simulink model "zawory_wyliczane"  (R2021b)
settings: Solver=VariableStepAuto  StartTime=0.0  StopTime=10.0  RelTol=1e-3
undefined symbols (not defined in the file): dpoN, dRz_b, dRz_g, dRz_p, Rb, Rg, Rk, Rp, RzN, skok_czas, zmiana_po
settings Model: Creator=adams  LastModifiedBy=adams

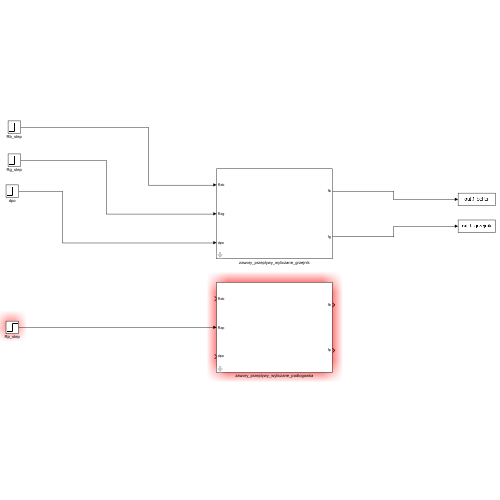
[thumbnail: Simulink's stored preview of the top-level diagram]
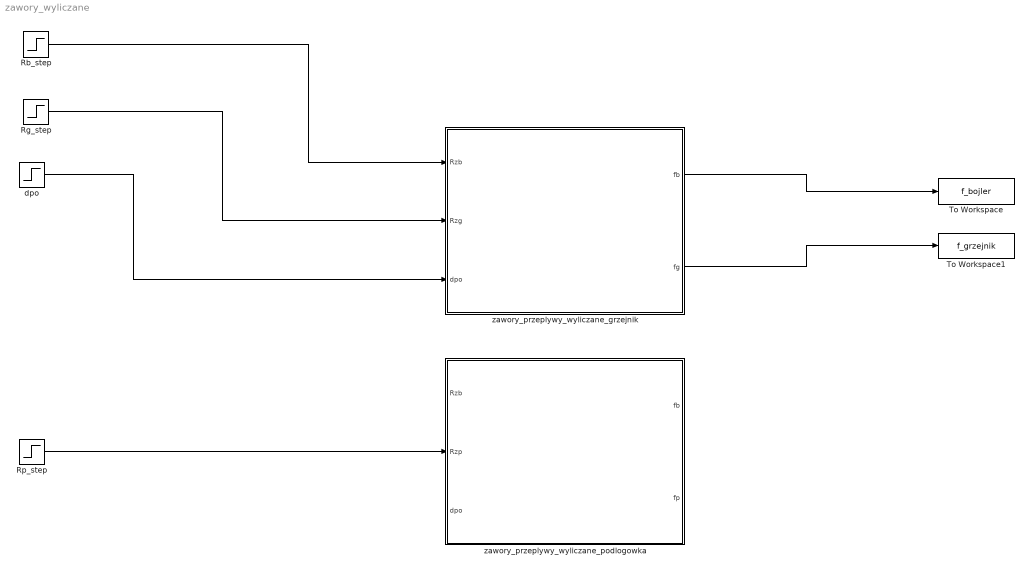
== system zawory_wyliczane ==
  Rb_step : Step  Time=skok_czas  Before=RzN  After=RzN + dRz_b  SampleTime=0
  Rg_step : Step  Time=skok_czas  Before=RzN  After=RzN + dRz_g  SampleTime=0
  Rp_step : Step  Time=skok_czas  Before=RzN  After=RzN + dRz_p  SampleTime=0
  To Workspace : ToWorkspace  VariableName=f_bojler  SampleTime=-1
  To Workspace1 : ToWorkspace  VariableName=f_grzejnik  SampleTime=-1
  dpo : Step  Time=skok_czas  Before=dpoN  After=dpoN + zmiana_po  SampleTime=0
  zawory_przeplywy_wyliczane_grzejnik : Subsystem  mask{Rk=Rk, Rb=Rb, Rg=Rg}
  zawory_przeplywy_wyliczane_podlogowka : Subsystem  mask{Rk=Rk, Rb=Rb, Rp=Rp}
  wires:
  Rb_step/1 -> zawory_przeplywy_wyliczane_grzejnik/1(Rzb)
  Rg_step/1 -> zawory_przeplywy_wyliczane_grzejnik/2(Rzg)
  dpo/1 -> zawory_przeplywy_wyliczane_grzejnik/3(dpo)
  zawory_przeplywy_wyliczane_grzejnik/1(fb) -> To Workspace/1
  zawory_przeplywy_wyliczane_grzejnik/2(fg) -> To Workspace1/1
  Rp_step/1 -> zawory_przeplywy_wyliczane_podlogowka/2(Rzp)

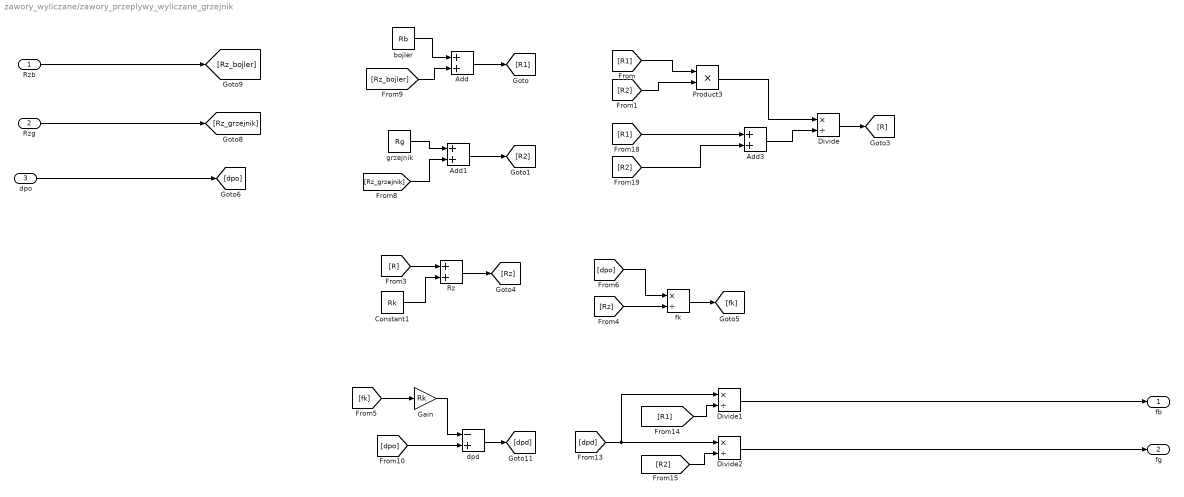
== system zawory_wyliczane/zawory_przeplywy_wyliczane_grzejnik ==
  Rzb : Inport
  Rzg : Inport  Port=2
  dpo : Inport  Port=3
  Add : Sum
  Add1 : Sum
  Add3 : Sum
  Constant1 : Constant  Value=Rk
  Divide : Product  Inputs=*/
  Divide1 : Product  Inputs=*/
  Divide2 : Product  Inputs=*/
  Gain : Gain  Gain=Rk
  Product3 : Product
  Rz : Sum
  bojler : Constant  Value=Rb
  dpd : Sum  Inputs=-+
  fk : Product  Inputs=*/
  grzejnik : Constant  Value=Rg
  fb : Outport
  fg : Outport  Port=2
  wires:
  Divide2/1 -> fg/1
  [R1] -> Add3/1
  [fk] -> Gain/1
  grzejnik/1 -> Add1/1
  Product3/1 -> Divide/1
  bojler/1 -> Add/1
  [R] -> Rz/1
  [R2] -> Add3/2
  Add3/1 -> Divide/2
  [R2] -> Product3/2
  [dpo] -> fk/1
  fk/1 -> [fk]
  [dpd] -> Divide2/1, Divide1/1
  [Rz_bojler] -> Add/2
  Add1/1 -> [R2]
  [R1] -> Divide1/2
  [R1] -> Product3/1
  Divide1/1 -> fb/1
  Constant1/1 -> Rz/2
  [R2] -> Divide2/2
  [Rz_grzejnik] -> Add1/2
  [dpo] -> dpd/2
  Rzg/1 -> [Rz_grzejnik]
  Gain/1 -> dpd/1
  Divide/1 -> [R]
  dpd/1 -> [dpd]
  Add/1 -> [R1]
  [Rz] -> fk/2
  Rz/1 -> [Rz]
  dpo/1 -> [dpo]
  Rzb/1 -> [Rz_bojler]

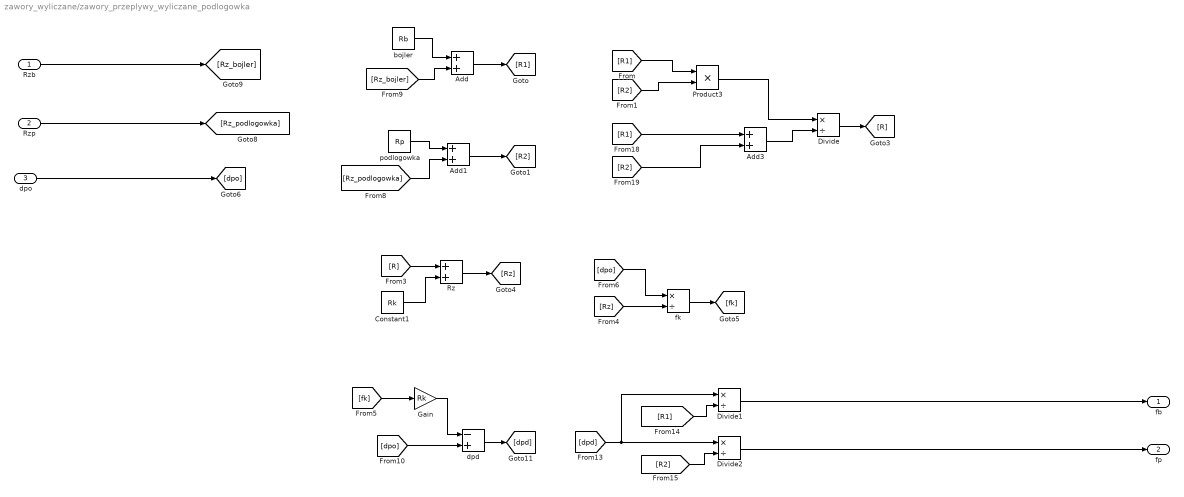
== system zawory_wyliczane/zawory_przeplywy_wyliczane_podlogowka ==
  Rzb : Inport
  Rzp : Inport  Port=2
  dpo : Inport  Port=3
  Add : Sum
  Add1 : Sum
  Add3 : Sum
  Constant1 : Constant  Value=Rk
  Divide : Product  Inputs=*/
  Divide1 : Product  Inputs=*/
  Divide2 : Product  Inputs=*/
  Gain : Gain  Gain=Rk
  Product3 : Product
  Rz : Sum
  bojler : Constant  Value=Rb
  dpd : Sum  Inputs=-+
  fk : Product  Inputs=*/
  podlogowka : Constant  Value=Rp
  fb : Outport
  fp : Outport  Port=2
  wires:
  Divide2/1 -> fp/1
  [R1] -> Add3/1
  [fk] -> Gain/1
  podlogowka/1 -> Add1/1
  Product3/1 -> Divide/1
  bojler/1 -> Add/1
  [R] -> Rz/1
  [R2] -> Add3/2
  Add3/1 -> Divide/2
  [R2] -> Product3/2
  [dpo] -> fk/1
  fk/1 -> [fk]
  [dpd] -> Divide2/1, Divide1/1
  [Rz_bojler] -> Add/2
  Add1/1 -> [R2]
  [R1] -> Divide1/2
  [R1] -> Product3/1
  Divide1/1 -> fb/1
  Constant1/1 -> Rz/2
  [R2] -> Divide2/2
  [Rz_podlogowka] -> Add1/2
  [dpo] -> dpd/2
  Rzp/1 -> [Rz_podlogowka]
  Gain/1 -> dpd/1
  Divide/1 -> [R]
  dpd/1 -> [dpd]
  Add/1 -> [R1]
  [Rz] -> fk/2
  Rz/1 -> [Rz]
  dpo/1 -> [dpo]
  Rzb/1 -> [Rz_bojler]
